simulink model "reentry_sim"  (R2016a)
settings: Solver=VariableStepAuto  StartTime=0.0  StopTime=4000  FixedStep=0.1  MaxStep=1  RelTol=1e-3
InitFcn:
  | init_conditions
values from neighbouring files (symbols this model uses):
  altitude_end = 2000    [init_conditions.m]
  AoA = 20    [init_conditions.m]
  atmo_data = importdata(atmo_filename)    [init_data.m]
  body_data = [body_data{row,2},body_data{row,3}]    [init_data.m]
  init_pos = [0;115000]    [init_conditions.m]
  init_vel = [3470;-100]    [init_conditions.m]
  mass = 39500    [init_conditions.m]
  vehicle_aerodata = [1.45,0.4,80.9]    [init_conditions.m]
libraries: simulink_lib x8, simulink_extras x1, simulink x1
settings Model: RequirementInfo={'linktype_rmi_simulink' 'simulink_lib' '' 'true' '' '' } %GIDa_6f06f984_84f3_4f44_828a_de2db4acfc80  Creator=Mario  LastModifiedBy=Mario
settings DataIOCC: FinalStateName=final_state  SaveOutput=off  SignalLogging=off  DSMLogging=off

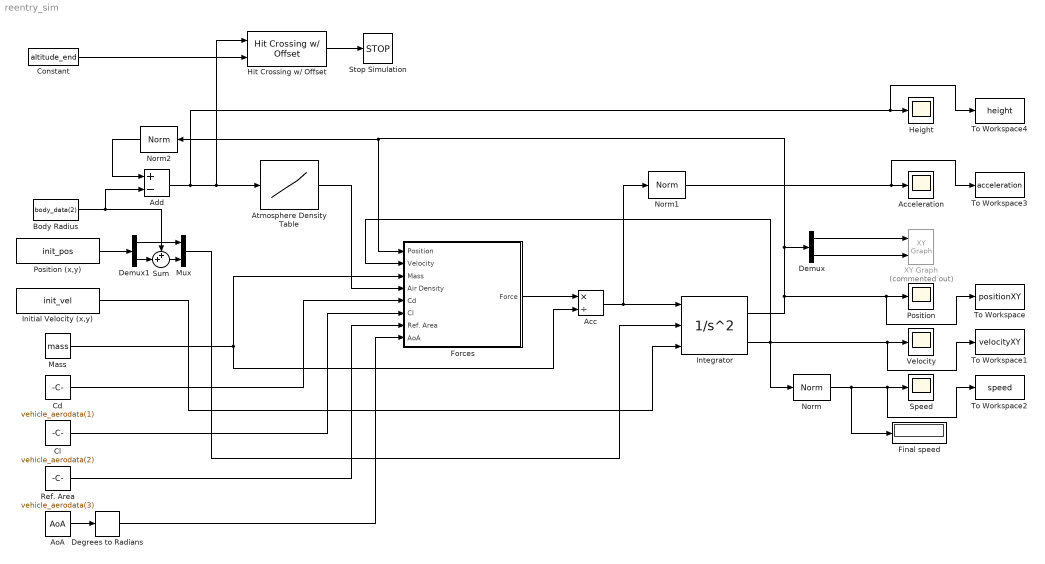
== system reentry_sim ==
  Acc : Product  Inputs=*/
  Acceleration : Scope
  Add : Sum  Inputs=+-
  AoA : Constant  Value=AoA
  Atmosphere Density Table : Lookup_n-D  NumberOfTableDimensions=1  BreakpointsForDimension1=atmo_data(:,1)  BreakpointsForDimension3=[5, 7]  Table=atmo_data(:,4)  InternalRulePriority=Speed  RndMeth=Simplest  InputSameDT=on
  Body Radius : Constant  Value=body_data(2)
  Cd : Constant  Value=vehicle_aerodata(1)
  Cl : Constant  Value=vehicle_aerodata(2)
  Constant : Constant  Value=altitude_end
  Degrees to Radians : simulink_extras/Transformations/Degrees to Radians
  Demux : Demux  Outputs=2
  Demux1 : Demux  Outputs=2
  Final speed : Display
  Forces : Subsystem
  Height : Scope
  Hit Crossing w/ Offset : simulink_lib/Hit Crossing w// Offset  direction=Falling
  Initial Velocity (x,y) : Constant  Value=init_vel
  Integrator : SecondOrderIntegrator  ICSourceX=external  ICSourceDXDT=external
  Mass : Constant  Value=mass
  Mux : Mux  Inputs=2
  Norm : simulink_lib/Norm
  Norm1 : simulink_lib/Norm
  Norm2 : simulink_lib/Norm
  Position : Scope
  Position (x,y) : Constant  Value=init_pos
  Ref. Area : Constant  Value=vehicle_aerodata(3)
  Speed : Scope
  Stop Simulation : Stop
  Sum : Sum  Inputs=++|
  To Workspace : ToWorkspace  VariableName=positionXY  SampleTime=-1
  To Workspace1 : ToWorkspace  VariableName=velocityXY  SampleTime=-1
  To Workspace2 : ToWorkspace  VariableName=speed  SampleTime=-1
  To Workspace3 : ToWorkspace  VariableName=acceleration  SampleTime=-1
  To Workspace4 : ToWorkspace  VariableName=height  SampleTime=-1
  Velocity : Scope
  XY Graph : simulink/Sinks/XY Graph  Commented=on  xmin=0  xmax=1.6e+6  ymin=3e+6  ymax=3.55e+6  st=-1
  wires:
  Position (x,y)/1 -> Demux1/1
  Initial Velocity (x,y)/1 -> Integrator/3
  Mass/1 -> Forces/3(Mass), Acc/2
  Norm2/1 -> Add/1
  Body Radius/1 -> Add/2, Sum/1
  Add/1 -> To Workspace4/1, Height/1, Hit Crossing w/ Offset/1, Atmosphere Density Table/1
  Atmosphere Density Table/1 -> Forces/4(Air Density)
  AoA/1 -> Degrees to Radians/1
  Ref. Area/1 -> Forces/7(Ref. Area)
  Degrees to Radians/1 -> Forces/8(AoA)
  Cd/1 -> Forces/5(Cd)
  Forces/1(Force) -> Acc/1
  Integrator/1 -> Demux/1, Norm2/1, Forces/1(Position), To Workspace/1, Position/1
  Demux/2 -> XY Graph/2
  Demux/1 -> XY Graph/1
  Norm/1 -> Final speed/1, To Workspace2/1, Speed/1
  Norm1/1 -> To Workspace3/1, Acceleration/1
  Acc/1 -> Norm1/1, Integrator/1
  Demux1/2 -> Sum/2
  Sum/1 -> Mux/2
  Demux1/1 -> Mux/1
  Mux/1 -> Integrator/2
  Integrator/2 -> Norm/1, Forces/2(Velocity), To Workspace1/1, Velocity/1
  Constant/1 -> Hit Crossing w/ Offset/2
  Hit Crossing w/ Offset/1 -> Stop Simulation/1
  Cl/1 -> Forces/6(Cl)

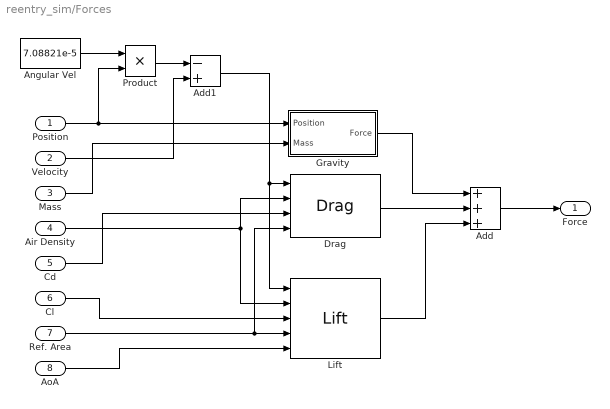
== system reentry_sim/Forces ==
  Position : Inport
  Velocity : Inport  Port=2
  Mass : Inport  Port=3
  Air Density : Inport  Port=4
  Cd : Inport  Port=5
  Cl : Inport  Port=6
  Ref. Area : Inport  Port=7
  AoA : Inport  Port=8
  Add : Sum  Inputs=3
  Add1 : Sum  Inputs=-+
  Angular Vel : Constant  Value=7.08821e-5
  Drag : simulink_lib/Drag  SystemSampleTime=-1
  Gravity : Subsystem  mask(Gravity){}
      mask help: Calculates gravitational force.
  Lift : simulink_lib/Lift  SystemSampleTime=-1
  Product : Product
  Force : Outport
  wires:
  Position/1 -> Gravity/1(Position), Product/2
  Mass/1 -> Gravity/2(Mass)
  Air Density/1 -> Drag/2, Lift/2
  Cd/1 -> Drag/3
  Cl/1 -> Lift/3
  Ref. Area/1 -> Drag/4, Lift/4
  AoA/1 -> Lift/5
  Gravity/1(Force) -> Add/1
  Drag/1 -> Add/2
  Lift/1 -> Add/3
  Add/1 -> Force/1
  Angular Vel/1 -> Product/1
  Product/1 -> Add1/1
  Velocity/1 -> Add1/2
  Add1/1 -> Drag/1, Lift/1

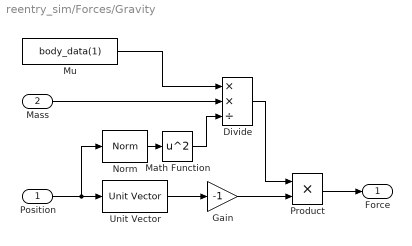
== system reentry_sim/Forces/Gravity ==
  Position : Inport
  Mass : Inport  Port=2
  Divide : Product  Inputs=**/  RndMeth=Round
  Gain : Gain  Gain=-1
  Math Function : Math  Operator=square  SaturateOnIntegerOverflow=on
  Mu : Constant  Value=body_data(1)
  Norm : simulink_lib/Unit Vector/Norm
  Product : Product
  Unit Vector : simulink_lib/Unit Vector
  Force : Outport
  wires:
  Math Function/1 -> Divide/3
  Norm/1 -> Math Function/1
  Divide/1 -> Product/1
  Product/1 -> Force/1
  Gain/1 -> Product/2
  Mass/1 -> Divide/2
  Mu/1 -> Divide/1
  Unit Vector/1 -> Gain/1
  Position/1 -> Unit Vector/1, Norm/1
